simulink library "lib_Conduction_InterfaceTemp"  (R2015a)
settings: Solver=ode45  StartTime=0.0  StopTime=10.0  RelTol=1e-3
libraries: lib_GenTools_WeightedAveraging x1
settings Model: Creator=jlkratz  LastModifiedBy=jlkratz

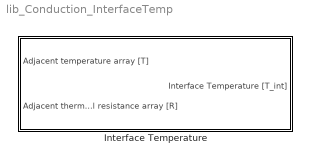
== system lib_Conduction_InterfaceTemp ==
  Interface Temperature : Subsystem  mask(TSAT: Interface Temperature Block){Int_horiz_M=off, Int_vert_M=off, Int_pt_M=on}
      mask prompts: Int_horiz_M "Int_horiz_M - The interface is a line that runs horizontally"; Int_vert_M "Int_vert_M - The interafce is a line that runs vertically"; Int_pt_M "Int_pt_M - The interface is a single point"
      mask help: This function is meant for estimating the temperature at an interface in a structure with multiple paths to transmit heat. This could be applicable to transitions in material or geometries in which various components connect together at the same location. Each connection to the interface has a temperature associated with it that is adjacent to the interface and a distance from the interface through which heat is conducted. The interface temperature is estimated using a weighted averaging technique based on the ratio of the thermal conductivity to the distance to the interface (k/L). The interface can be treated as a line or a point.
      mask init:
      | %set parameters
      | 
      | delete_line(gcb,'Weighted Averaging/1','Interface Temperature [T_int]/1')
      | set_param([gcb,'/Weighted Averaging'],'avg_cols_M',Int_horiz_M);
      | set_param([gcb,'/Weighted Averaging'],'avg_rows_M',Int_vert_M);
      | set_param([gcb,'/Weighted Averaging'],'avg_all_M',Int_pt_M);
      | add_line(gcb,'Weighted Averaging/1','Interface Temperature [T_int]/1','autorouting','on')
      mask Help: web(which('Conduction_TSAT_InterfaceTemp.html'),'-helpbrowser')
      mask Callback Int_horiz_M:
      | if length(get_param(gcb,'Int_horiz_M')) == 2 %on
      |     set_param(gcb,'Int_vert_M','off');
      |     set_param(gcb,'Int_pt_M','off');
      | end
      mask Callback Int_vert_M:
      | if length(get_param(gcb,'Int_vert_M')) == 2 %on
      |     set_param(gcb,'Int_horiz_M','off');
      |     set_param(gcb,'Int_pt_M','off');
      | end
      mask Callback Int_pt_M:
      | if length(get_param(gcb,'Int_pt_M')) == 2 %on
      |     set_param(gcb,'Int_vert_M','off');
      |     set_param(gcb,'Int_horiz_M','off');
      | end
      mask DialogControl Container3 Prompt: Interface Type

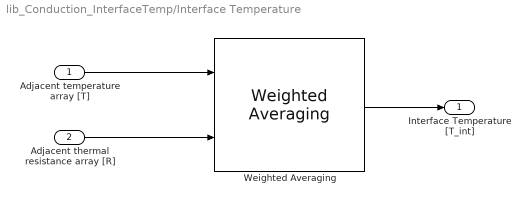
== system lib_Conduction_InterfaceTemp/Interface Temperature ==
  Adjacent temperature array [T] : Inport
  Adjacent thermal resistance array [R] : Inport  Port=2
  Weighted Averaging : lib_GenTools_WeightedAveraging/Weighted Averaging  avg_rows_M=off  avg_cols_M=off  avg_all_M=on  BN_M=gcb
  Interface Temperature [T_int] : Outport
  wires:
  Adjacent temperature array [T]/1 -> Weighted Averaging/1
  Adjacent thermal resistance array [R]/1 -> Weighted Averaging/2
  Weighted Averaging/1 -> Interface Temperature [T_int]/1
